simulink model "IfCase"  (R2015a)
settings: Solver=ode45  SolverMode=SingleTasking  StartTime=0.0  StopTime=10.0  RelTol=1e-3
settings Model: CovMetricSettings=dwe  CovHtmlReporting=off  covSaveCumulativeToWorkspaceVar=off  CovSaveSingleToWorkspaceVar=off  CovExternalEMLEnable=on  Creator=hbourbou  LastModifiedBy=hbourbou
settings DataIOCC: LimitDataPoints=off  SaveFormat=Dataset
settings DebuggingCC: SFUnexpectedBacktrackingDiag=error  SFNoUnconditionalDefaultTransitionDiag=error
settings HardwareCC: ProdBitPerPointer=64  ProdLargestAtomicFloat=Float  ProdIntDivRoundTo=Zero  ProdEndianess=LittleEndian  ProdHWDeviceType=Specified
settings ModelReferenceCC: PropagateSignalLabelsOutOfModel=on
settings GRTTargetCC: TargetLangStandard=C99 (ISO)  GeneratePreprocessorConditionals=Use local settings

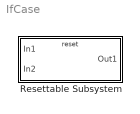
== system IfCase ==
  Resettable Subsystem : Subsystem  TreatAsAtomicUnit=on

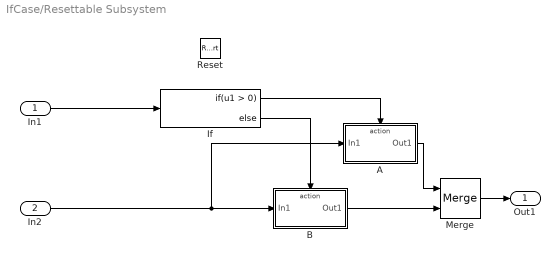
== system IfCase/Resettable Subsystem ==
  In1 : Inport
  In2 : Inport  Port=2
  Reset : ResetPort  DisableCoverage=on
  A : Subsystem  TreatAsAtomicUnit=on
  B : Subsystem  TreatAsAtomicUnit=on
  If : If
  Merge : Merge
  Out1 : Outport
  wires:
  In1/1 -> If/1
  If/1 -> A/Action
  If/2 -> B/Action
  In2/1 -> A/1(In1), B/1(In1)
  Merge/1 -> Out1/1
  A/1(Out1) -> Merge/1
  B/1(Out1) -> Merge/2

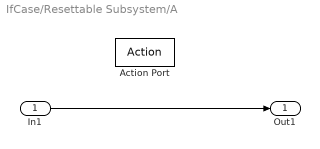
== system IfCase/Resettable Subsystem/A ==
  In1 : Inport
  Action Port : ActionPort  ActionType=then
  Out1 : Outport
  wires:
  In1/1 -> Out1/1

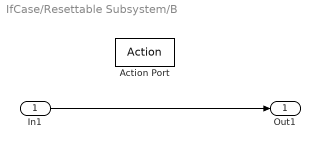
== system IfCase/Resettable Subsystem/B ==
  In1 : Inport
  Action Port : ActionPort  ActionType=else
  Out1 : Outport
  wires:
  In1/1 -> Out1/1
